simulink model "EulerWheel"  (R2019b)
settings: Solver=ode113  StartTime=0.0  StopTime=SimTime  MinStep=1e-10  RelTol=1e-15  AbsTol=1e-19
values from neighbouring files (symbols this model uses):
  I = diag( [I_x I_y I_z ] )    [Lab_3.m]    (also in Lab_5.m)
  I_inv = inv( I )    [Lab_3.m]    (also in Lab_5.m)
  I_z = 0.0109    [Lab_3.m]    (also in Lab_5.m)
  Iw = 0.005    [Lab_3.m]
  w_0 = [1e-6 1e-6 0.02]    [Lab_3.m]    (also in Lab_5.m = [ w_0x w_0y w_0z ])
settings Model: Creator=adity  LastModifiedBy=adity

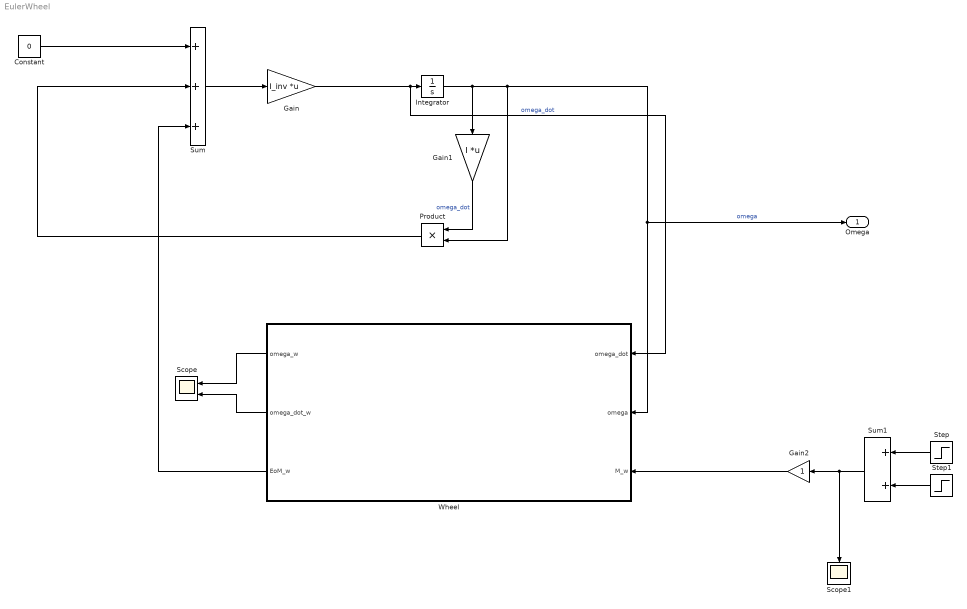
== system EulerWheel ==
  Constant : Constant  Value=0
  Gain : Gain  Gain=I_inv  Multiplication=Matrix(K*u) (u vector)
  Gain1 : Gain  Gain=I  Multiplication=Matrix(K*u) (u vector)
  Gain2 : Gain
  Integrator : Integrator  InitialCondition=w_0  AbsoluteTolerance=1e-19
  Product : Product
  Scope : Scope  NumInputPorts=2
  Scope1 : Scope
  Step : Step  Time=0  SampleTime=0
  Step1 : Step  Time=0.1  Before=1  After=0  SampleTime=0
  Sum : Sum  Inputs=+++
  Sum1 : Sum
  Wheel : Subsystem
  Omega : Outport
  wires:
  Wheel/3(EoM_w) -> Sum/3
  Sum/1 -> Gain/1
  Gain/1 -> Wheel/1(omega_dot), Integrator/1  "omega_dot"
  Integrator/1 -> Product/2, Omega/1, Wheel/2(omega), Gain1/1  "omega"
  Gain1/1 -> Product/1  "omega_dot"
  Product/1 -> Sum/2
  Wheel/1(omega_w) -> Scope/1
  Wheel/2(omega_dot_w) -> Scope/2
  Constant/1 -> Sum/1
  Step/1 -> Sum1/1
  Step1/1 -> Sum1/2
  Sum1/1 -> Gain2/1, Scope1/1
  Gain2/1 -> Wheel/3(M_w)

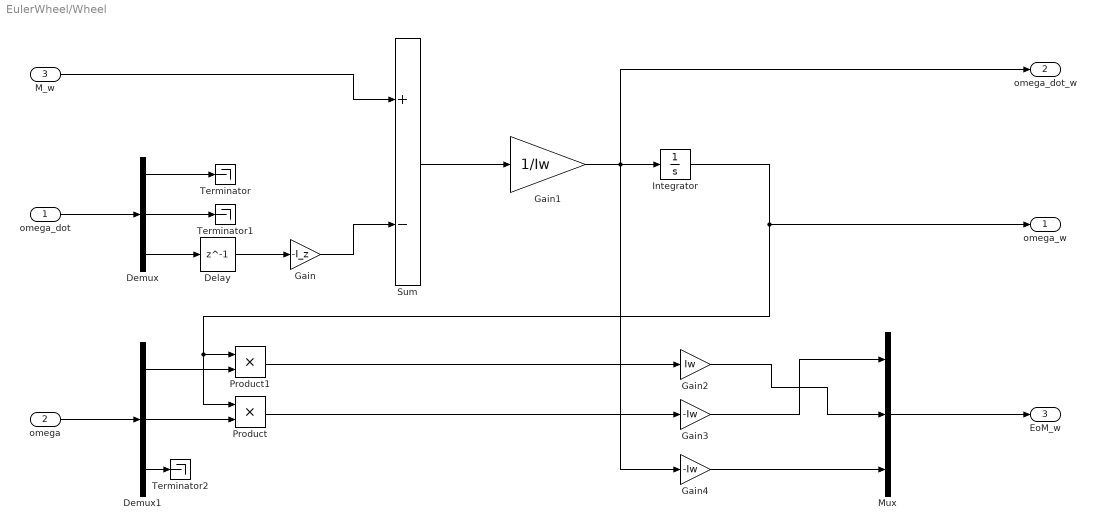
== system EulerWheel/Wheel ==
  omega_dot : Inport
  omega : Inport  Port=2
  M_w : Inport  Port=3
  Delay : Delay  DelayLength=1
  Demux : Demux  Outputs=3
  Demux1 : Demux  Outputs=3
  Gain : Gain  Gain=-I_z
  Gain1 : Gain  Gain=1/Iw
  Gain2 : Gain  Gain=Iw
  Gain3 : Gain  Gain=-Iw
  Gain4 : Gain  Gain=-Iw
  Integrator : Integrator
  Mux : Mux  Inputs=3
  Product : Product
  Product1 : Product
  Sum : Sum  Inputs=+-
  Terminator : Terminator
  Terminator1 : Terminator
  Terminator2 : Terminator
  omega_w : Outport
  omega_dot_w : Outport  Port=2
  EoM_w : Outport  Port=3
  wires:
  omega_dot/1 -> Demux/1
  Demux/2 -> Terminator1/1
  Demux/1 -> Terminator/1
  Demux/3 -> Delay/1
  Gain/1 -> Sum/2
  M_w/1 -> Sum/1
  Sum/1 -> Gain1/1
  Gain1/1 -> omega_dot_w/1, Gain4/1, Integrator/1
  omega/1 -> Demux1/1
  Demux1/3 -> Terminator2/1
  Integrator/1 -> Product1/1, Product/1, omega_w/1
  Demux1/2 -> Product/2
  Demux1/1 -> Product1/2
  Product1/1 -> Gain2/1
  Product/1 -> Gain3/1
  Gain4/1 -> Mux/3
  Gain3/1 -> Mux/1
  Gain2/1 -> Mux/2
  Mux/1 -> EoM_w/1
  Delay/1 -> Gain/1
